simulink model "open_loop_control"  (Simulink 10.0)
settings: Solver=ode45  StartTime=0.0  StopTime=20.0  RelTol=1e-3  EnableMultiTasking=on
settings Model: Creator=akari  LastModifiedBy=linesLK
settings DataIOCC: LimitDataPoints=on  SignalLoggingSaveFormat=ModelDataLogs
settings OptimizationCC: ExpressionDepthLimit=2147483647
settings DebuggingCC: FcnCallInpInsideContextMsg=warning  StateNameClashWarn=warning
settings ConfigComp: CovExternalEMLEnable=off

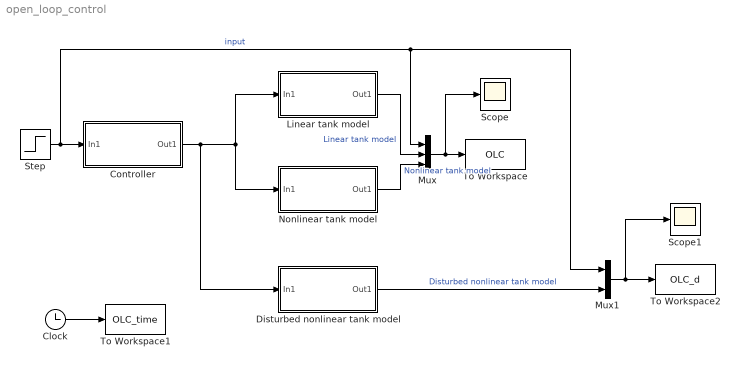
== system open_loop_control ==
  Clock : Clock
  Controller : Subsystem
  Disturbed nonlinear tank model : Subsystem
  Linear tank model : Subsystem
  Mux : Mux  Inputs=3
  Mux1 : Mux  Inputs=2
  Nonlinear tank model : Subsystem
  Scope : Scope
  Scope1 : Scope
  Step : Step  Time=10  Before=0.6  After=1.8  SampleTime=0
  To Workspace : ToWorkspace  VariableName=OLC  SampleTime=-1
  To Workspace1 : ToWorkspace  VariableName=OLC_time  SampleTime=-1
  To Workspace2 : ToWorkspace  VariableName=OLC_d  SampleTime=-1
  wires:
  Controller/1(Out1) -> Linear tank model/1(In1), Nonlinear tank model/1(In1), Disturbed nonlinear tank model/1(In1)
  Mux/1 -> To Workspace/1, Scope/1
  Step/1 -> Controller/1(In1), Mux/1, Mux1/1  "input"
  Clock/1 -> To Workspace1/1
  Nonlinear tank model/1(Out1) -> Mux/3  "Nonlinear tank model"
  Linear tank model/1(Out1) -> Mux/2  "Linear tank model"
  Mux1/1 -> To Workspace2/1, Scope1/1
  Disturbed nonlinear tank model/1(Out1) -> Mux1/2  "Disturbed nonlinear tank model"

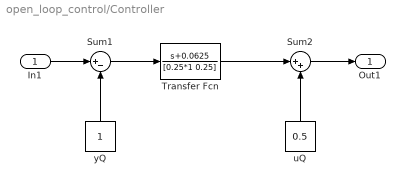
== system open_loop_control/Controller ==
  In1 : Inport
  Sum1 : Sum  Inputs=|+-
  Sum2 : Sum  Inputs=|++
  Transfer Fcn : TransferFcn  Numerator=[1 0.0625]  Denominator=[0.25*1 0.25]
  uQ : Constant  Value=0.5
  yQ : Constant
  Out1 : Outport
  wires:
  Sum1/1 -> Transfer Fcn/1
  Transfer Fcn/1 -> Sum2/1
  Sum2/1 -> Out1/1
  In1/1 -> Sum1/1
  yQ/1 -> Sum1/2
  uQ/1 -> Sum2/2

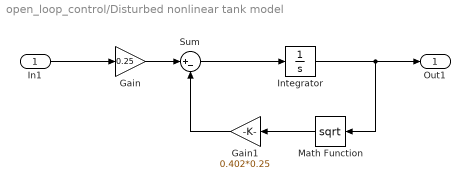
== system open_loop_control/Disturbed nonlinear tank model ==
  In1 : Inport
  Gain : Gain  Gain=0.25
  Gain1 : Gain  Gain=0.402*0.25
  Integrator : Integrator  InitialCondition=1
  Math Function : Math  Operator=sqrt  SaturateOnIntegerOverflow=on
  Sum : Sum  Inputs=|+-
  Out1 : Outport
  wires:
  Sum/1 -> Integrator/1
  Integrator/1 -> Math Function/1, Out1/1
  Math Function/1 -> Gain1/1
  Gain/1 -> Sum/1
  Gain1/1 -> Sum/2
  In1/1 -> Gain/1

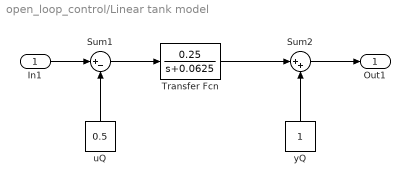
== system open_loop_control/Linear tank model ==
  In1 : Inport
  Sum1 : Sum  Inputs=|+-
  Sum2 : Sum  Inputs=|++
  Transfer Fcn : TransferFcn  Numerator=[0.25]  Denominator=[1 0.0625]
  uQ : Constant  Value=0.5
  yQ : Constant
  Out1 : Outport
  wires:
  Sum1/1 -> Transfer Fcn/1
  Transfer Fcn/1 -> Sum2/1
  yQ/1 -> Sum2/2
  uQ/1 -> Sum1/2
  Sum2/1 -> Out1/1
  In1/1 -> Sum1/1

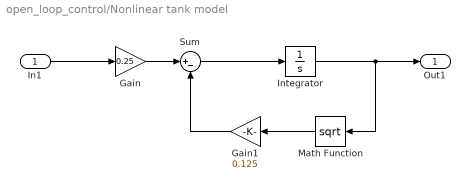
== system open_loop_control/Nonlinear tank model ==
  In1 : Inport
  Gain : Gain  Gain=0.25
  Gain1 : Gain  Gain=0.125
  Integrator : Integrator  InitialCondition=1
  Math Function : Math  Operator=sqrt  SaturateOnIntegerOverflow=on
  Sum : Sum  Inputs=|+-
  Out1 : Outport
  wires:
  Sum/1 -> Integrator/1
  Integrator/1 -> Math Function/1, Out1/1
  Math Function/1 -> Gain1/1
  Gain/1 -> Sum/1
  Gain1/1 -> Sum/2
  In1/1 -> Gain/1
